simulink model "Regler"  (R2021b)
settings: Solver=VariableStepAuto  StartTime=0.0  StopTime=10.0  RelTol=1e-3
model workspace (MAT data in the model file):
  D = Simulink.Parameter
  D.Value = [0 0.1 1]
  D.DataType = 'auto'
  D.Complexity = 'real'
  D.Dimensions = [1 3]
  Kr = Simulink.Parameter
  Kr.Value = 0.65
  Kr.DataType = 'auto'
  Kr.Complexity = 'real'
  Kr.Dimensions = [1 1]
  N = Simulink.Parameter
  N.Value = [0.9 1]
  N.DataType = 'auto'
  N.Complexity = 'real'
  N.Dimensions = [1 2]
settings Model: ParameterArgumentNames=Kr,N,D  Creator=Hoorsana  LastModifiedBy=Hoorsana

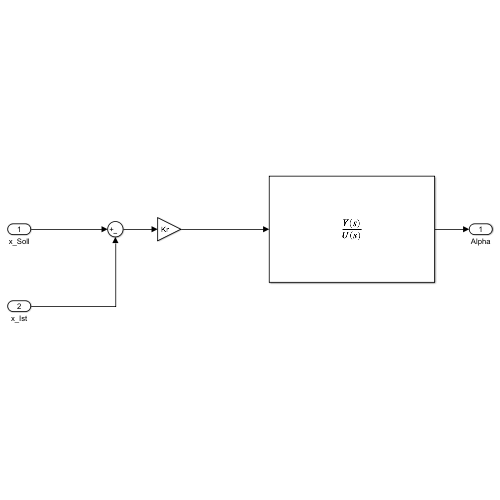
[thumbnail: Simulink's stored preview of the top-level diagram]
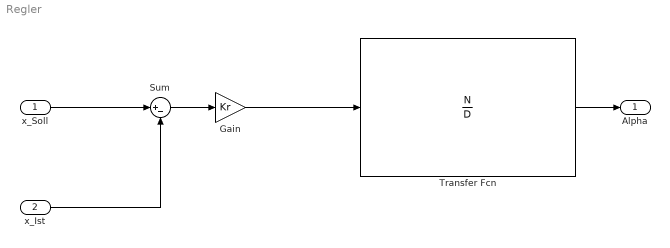
== system Regler ==
  x_Soll : Inport
  x_Ist : Inport  Port=2
  Gain : Gain  Gain=Kr
  Sum : Sum  Inputs=|+-
  Transfer Fcn : TransferFcn  Numerator=N  Denominator=D
  Alpha : Outport  VectorParamsAs1DForOutWhenUnconnected=off
  wires:
  Transfer Fcn/1 -> Alpha/1
  Sum/1 -> Gain/1
  Gain/1 -> Transfer Fcn/1
  x_Soll/1 -> Sum/1
  x_Ist/1 -> Sum/2
